simulink model "pendulum_friction_coefficient_identification_model"  (R2024b)
settings: Solver=FixedStepAuto  StartTime=0.0  StopTime=T1(end)  FixedStep=0.01  RelTol=1e-3
values from neighbouring files (symbols this model uses):
  fi0 = -1.56511504441    [currwork.mat]    (also in pendulum_friction_coefficient_identification.m = angle(1))
  g = 9.81    [currwork.mat]    (also in pendulum_friction_coefficient_identification.m)
  J_pend = 0.026668518142893    (= 0.0266685181429)    [pendulum_friction_coefficient_identification.m]
  omega0 = 422.554608411    [currwork.mat]    (also in pendulum_friction_coefficient_identification.m = 0)
  U = 0.012144    [currwork.mat]    (also in pendulum_friction_coefficient_identification.m)
  uc_init = 0.001    [currwork.mat]    (also in pendulum_friction_coefficient_identification.m)
  uv_init = 0.001    [currwork.mat]    (also in pendulum_friction_coefficient_identification.m)
settings Model: Creator=Student  LastModifiedBy=Paweł Wiktor
settings SolverCC: AlgebraicLoopSolver=TrustRegion
settings DataIOCC: ReturnWorkspaceOutputs=off
settings DebuggingCC: UnconnectedInputMsg=warning  UnconnectedOutputMsg=warning  UnconnectedLineMsg=warning  ArithmeticOperatorsInVariantConditions=warning
settings ModelReferenceCC: EnableRefExpFcnMdlSchedulingChecks=on
settings SFSimCC: CustomCodeUndefinedFunction=UseInterfaceOnly
settings RTWCC: GPUComputeCapability=3.5

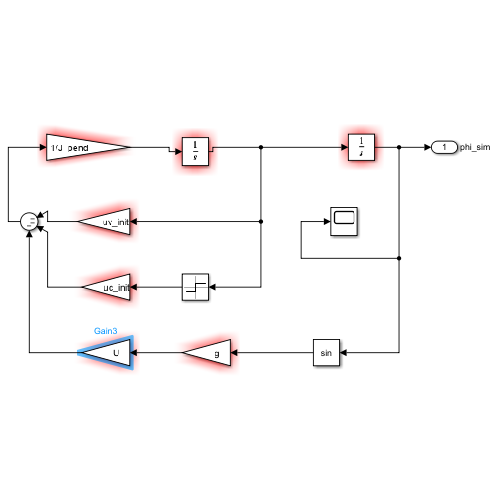
[thumbnail: Simulink's stored preview of the top-level diagram]
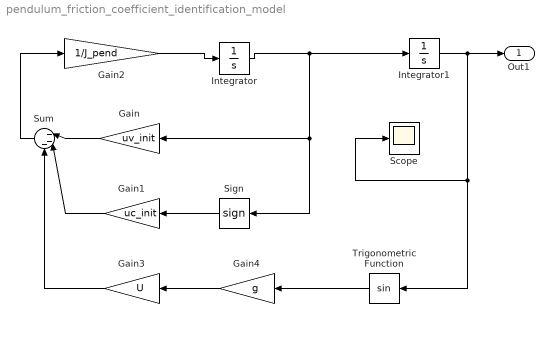
== system pendulum_friction_coefficient_identification_model ==
  Gain : Gain  Gain=uv_init
  Gain1 : Gain  Gain=uc_init
  Gain2 : Gain  Gain=1/J_pend
  Gain3 : Gain  Gain=U
  Gain4 : Gain  Gain=g
  Integrator : Integrator  InitialCondition=omega0
  Integrator1 : Integrator  InitialCondition=fi0
  Scope : Scope
  Sign : Signum  ZeroCross=off
  Sum : Sum  Inputs=|---
  Trigonometric Function : Trigonometry
  Out1 : Outport  SignalName=phi_sim  VectorParamsAs1DForOutWhenUnconnected=off
  wires:
  Gain2/1 -> Integrator/1
  Gain1/1 -> Sum/2
  Gain/1 -> Sum/1
  Integrator/1 -> Gain/1, Sign/1, Integrator1/1
  Sign/1 -> Gain1/1
  Sum/1 -> Gain2/1
  Integrator1/1 -> Scope/1, Trigonometric Function/1, Out1/1
  Gain4/1 -> Gain3/1
  Gain3/1 -> Sum/3
  Trigonometric Function/1 -> Gain4/1
